simulink model "sampleModel1734_sub"  (R2023a)
settings: Solver=VariableStepAuto  StartTime=0.0  StopTime=10.0  RelTol=1e-3
libraries: hdlsllib x3
settings Model: Creator=user1  LastModifiedBy=user1
settings OptimizationCC: BlockReduction=off  ConditionallyExecuteInputs=off

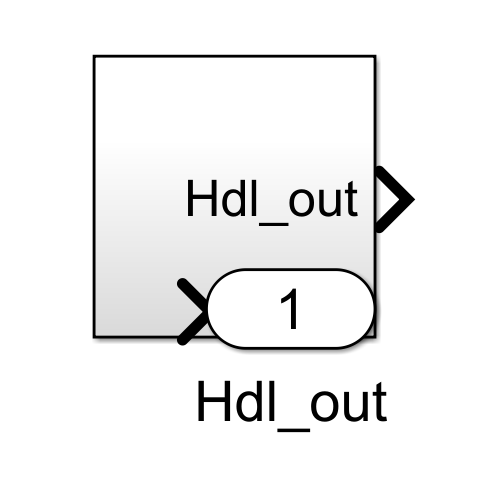
[thumbnail: Simulink's stored preview of the top-level diagram]
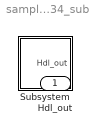
== system sampleModel1734_sub ==
  Subsystem : Subsystem
  Hdl_out : Outport  OutDataTypeStr=uint8

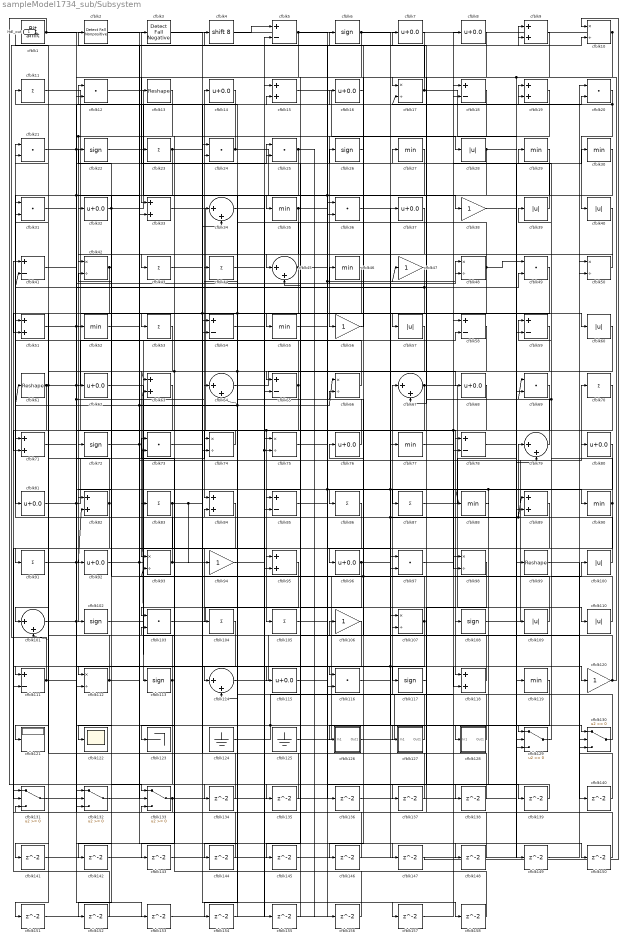
== system sampleModel1734_sub/Subsystem ==
  cfblk1 : hdlsllib/Logic and Bit Operations/Bit Shift  mode=Shift Left Logical  N=0
  cfblk{10,17,42,48,50,66,74..75,93,98,107,112} (12 alike) : Product  Inputs=*/  OutDataTypeStr=uint8  RndMeth=Zero  SaturateOnIntegerOverflow=on
  cfblk{28,39..40,57,60,100,109..110} (8 alike) : Abs  OutDataTypeStr=uint8  SaturateOnIntegerOverflow=off
  cfblk{34,45,64,67,79,101,114} (7 alike) : Sum  Inputs=|++  OutDataTypeStr=uint8
  cfblk{6,22,26,72,102,108,113,117} (8 alike) : Signum
  cfblk{12,20..21,24..25,31,36,49,69,73,97,103,116} (13 alike) : DotProduct  OutDataTypeStr=uint8
  cfblk{11,23,43..44,53,70,83,86..87,91,104..105} (12 alike) : Sum  Inputs=+  OutDataTypeStr=uint8
  cfblk{38,47,56,94,106,120} (6 alike) : Gain  OutDataTypeStr=uint8
  cfblk{5,18,41,54,58..59,65,78,85,111} (10 alike) : Sum  Inputs=+-  OutDataTypeStr=uint8
  cfblk{7..8,14,16,32,37,62,68,76,80..81,92,96,115} (14 alike) : Bias  Bias=0.0  SaturateOnIntegerOverflow=off
  cfblk{9,15,19,33,51,63,71,82,84,89,95,118} (12 alike) : Sum  OutDataTypeStr=uint8
  cfblk{27,29..30,35,46,52,55,77,88,90,119} (11 alike) : MinMax  OutDataTypeStr=uint8
  cfblk121 : Display
  cfblk122 : Scope
  cfblk123 : Terminator
  cfblk124 : Ground
  cfblk125 : Ground
  cfblk126 : Subsystem
      settings: LibrarySourceBlock=|
      | hdlsllib/Ports &
      | Subsystems/Subsystem
  cfblk127 : Subsystem
      settings: LibrarySourceBlock=|
      | hdlsllib/Ports &
      | Subsystems/Subsystem
  cfblk128 : Subsystem
      settings: LibrarySourceBlock=|
      | hdlsllib/Ports &
      | Subsystems/Subsystem
  cfblk{129..133} (5 alike) : Switch  OutDataTypeStr=uint8  SaturateOnIntegerOverflow=off  InputSameDT=off
  cfblk13 : Reshape
  cfblk{134..158} (25 alike) : Delay  SampleTime=1
  cfblk2 : hdlsllib/Logic and Bit Operations/Detect Fall Nonpositive  vinit=0  OutDataTypeStr=uint8
  cfblk3 : hdlsllib/Logic and Bit Operations/Detect Fall Negative  vinit=0  OutDataTypeStr=uint8
  cfblk4 : ArithShift  BitShiftNumber=8
  cfblk61 : Reshape
  cfblk99 : Reshape
  Hdl_out : Outport  OutDataTypeStr=uint8
  wires:
  cfblk100/1 -> cfblk42/2, cfblk79/1
  cfblk69/1 -> cfblk85/2, cfblk105/1
  cfblk89/1 -> cfblk91/1
  cfblk12/1 -> cfblk38/1
  cfblk63/1 -> cfblk102/1
  cfblk59/1 -> cfblk154/1, cfblk113/1
  cfblk13/1 -> cfblk72/1
  cfblk66/1 -> cfblk14/1
  cfblk108/1 -> cfblk70/1
  cfblk120/1 -> cfblk25/2, cfblk17/1
  cfblk15/1 -> cfblk28/1
  cfblk11/1 -> cfblk55/1
  cfblk67/1 -> cfblk122/1, cfblk110/1
  cfblk32/1 -> cfblk52/1, cfblk16/1
  cfblk96/1 -> cfblk135/1, cfblk130/3
  cfblk111/1 -> cfblk15/2, cfblk4/1
  cfblk130/1 -> cfblk67/1
  cfblk21/1 -> cfblk115/1, cfblk118/1
  cfblk46/1 -> cfblk53/1
  cfblk38/1 -> cfblk99/1
  cfblk64/1 -> cfblk68/1
  cfblk14/1 -> cfblk132/3, cfblk32/1
  cfblk110/1 -> cfblk39/1, cfblk69/1
  cfblk9/1 -> cfblk129/3, cfblk86/1
  cfblk65/1 -> cfblk31/2, cfblk84/1
  cfblk1/1 -> cfblk133/1, cfblk33/2, cfblk130/1
  cfblk26/1 -> cfblk96/1
  cfblk33/1 -> cfblk78/1
  cfblk62/1 -> cfblk117/1
  cfblk109/1 -> cfblk22/1
  cfblk81/1 -> cfblk83/1, cfblk34/1
  cfblk116/1 -> cfblk48/2, cfblk89/1
  cfblk50/1 -> cfblk45/1
  cfblk22/1 -> cfblk24/2
  cfblk93/1 -> cfblk157/1, cfblk21/1
  cfblk103/1 -> cfblk108/1
  cfblk18/1 -> cfblk56/1
  cfblk76/1 -> cfblk44/1
  cfblk71/1 -> cfblk64/1
  cfblk54/1 -> cfblk120/1, cfblk75/2
  cfblk23/1 -> cfblk158/1, cfblk81/1
  cfblk19/1 -> cfblk103/1
  cfblk17/1 -> cfblk109/1, cfblk2/1
  cfblk51/1 -> cfblk78/2, cfblk74/1
  cfblk37/1 -> cfblk42/1
  cfblk56/1 -> cfblk6/1
  cfblk92/1 -> cfblk19/2, cfblk34/2
  cfblk27/1 -> cfblk35/1
  cfblk53/1 -> cfblk82/1
  cfblk86/1 -> cfblk104/1
  cfblk20/1 -> cfblk17/2, cfblk40/1
  cfblk117/1 -> cfblk7/1
  cfblk125/1 -> cfblk8/1
  cfblk79/1 -> cfblk26/1
  cfblk101/1 -> cfblk148/1, cfblk46/1
  cfblk41/1 -> cfblk25/1
  cfblk90/1 -> cfblk92/1, cfblk27/1
  cfblk39/1 -> cfblk3/1
  cfblk57/1 -> cfblk93/1
  cfblk102/1 -> cfblk106/1
  cfblk126/1(Out1) -> cfblk98/1
  cfblk4/1 -> cfblk5/1
  cfblk2/1 -> cfblk95/1
  cfblk87/1 -> cfblk30/1
  cfblk82/1 -> cfblk21/2, cfblk121/1
  cfblk61/1 -> cfblk71/2, cfblk101/2, cfblk147/1, cfblk37/1
  cfblk42/1 -> cfblk62/1, cfblk111/1
  cfblk95/1 -> cfblk123/1
  cfblk36/1 -> cfblk107/1
  cfblk10/1 -> Hdl_out/1, cfblk65/1
  cfblk45/1 -> cfblk13/1, cfblk51/2, cfblk19/1
  cfblk128/1(Out1) -> cfblk61/1, cfblk64/2
  cfblk97/1 -> cfblk10/2
  cfblk16/1 -> cfblk116/1
  cfblk132/1 -> cfblk80/1
  cfblk127/1(Out1) -> cfblk11/1
  cfblk52/1 -> cfblk90/1
  cfblk94/1 -> cfblk48/1
  cfblk72/1 -> cfblk150/1, cfblk66/1, cfblk9/1
  cfblk114/1 -> cfblk50/2
  cfblk80/1 -> cfblk128/1(In1), cfblk116/2
  cfblk113/1 -> cfblk152/1, cfblk31/1
  cfblk28/1 -> cfblk142/1, cfblk119/1
  cfblk119/1 -> cfblk126/1(In1)
  cfblk91/1 -> cfblk82/2, cfblk49/2, cfblk63/2
  cfblk35/1 -> cfblk129/1, cfblk43/1
  cfblk70/1 -> cfblk132/2, cfblk98/2
  cfblk129/1 -> cfblk59/1
  cfblk133/1 -> cfblk131/3, cfblk18/1
  cfblk124/1 -> cfblk129/2, cfblk58/1
  cfblk49/1 -> cfblk144/1, cfblk143/1, cfblk63/1
  cfblk29/1 -> cfblk67/2
  cfblk77/1 -> cfblk29/1
  cfblk105/1 -> cfblk9/2, cfblk47/1
  cfblk118/1 -> cfblk76/1
  cfblk73/1 -> cfblk20/2
  cfblk3/1 -> cfblk87/1
  cfblk30/1 -> cfblk95/2
  cfblk106/1 -> cfblk111/2
  cfblk131/1 -> cfblk73/1
  cfblk5/1 -> cfblk12/2, cfblk139/1, cfblk88/1
  cfblk48/1 -> cfblk145/1, cfblk49/1, cfblk12/1
  cfblk44/1 -> cfblk5/2
  cfblk47/1 -> cfblk41/2, cfblk85/1
  cfblk7/1 -> cfblk33/1
  cfblk8/1 -> cfblk57/1
  cfblk83/1 -> cfblk112/2, cfblk94/1, cfblk74/2
  cfblk24/1 -> cfblk23/1, cfblk77/1, cfblk36/2
  cfblk75/1 -> cfblk97/2
  cfblk6/1 -> cfblk54/2, cfblk89/2, cfblk118/2, cfblk130/2
  cfblk25/1 -> cfblk156/1, cfblk114/1
  cfblk74/1 -> cfblk71/1
  cfblk55/1 -> cfblk60/1
  cfblk107/1 -> cfblk112/1, cfblk93/2, cfblk66/2
  cfblk112/1 -> cfblk51/1, cfblk100/1
  cfblk60/1 -> cfblk101/1
  cfblk84/1 -> cfblk131/2
  cfblk43/1 -> cfblk59/2, cfblk127/1(In1)
  cfblk115/1 -> cfblk58/2
  cfblk40/1 -> cfblk134/1
  cfblk134/1 -> cfblk1/1
  cfblk135/1 -> cfblk24/1
  cfblk85/1 -> cfblk136/1
  cfblk136/1 -> cfblk69/2
  cfblk98/1 -> cfblk137/1
  cfblk137/1 -> cfblk84/2
  cfblk88/1 -> cfblk138/1
  cfblk138/1 -> cfblk54/1
  cfblk139/1 -> cfblk133/2
  cfblk99/1 -> cfblk140/1
  cfblk140/1 -> cfblk20/1
  cfblk58/1 -> cfblk141/1
  cfblk141/1 -> cfblk97/1
  cfblk142/1 -> cfblk15/1
  cfblk143/1 -> cfblk65/2
  cfblk144/1 -> cfblk103/2
  cfblk145/1 -> cfblk79/2
  cfblk68/1 -> cfblk146/1
  cfblk146/1 -> cfblk132/1
  cfblk147/1 -> cfblk10/1
  cfblk148/1 -> cfblk107/2
  cfblk78/1 -> cfblk149/1
  cfblk149/1 -> cfblk50/1
  cfblk150/1 -> cfblk41/1
  cfblk104/1 -> cfblk151/1
  cfblk151/1 -> cfblk75/1
  cfblk152/1 -> cfblk131/1
  cfblk31/1 -> cfblk153/1
  cfblk153/1 -> cfblk36/1
  cfblk154/1 -> cfblk114/2
  cfblk34/1 -> cfblk155/1
  cfblk155/1 -> cfblk45/2
  cfblk156/1 -> cfblk133/3
  cfblk157/1 -> cfblk18/2
  cfblk158/1 -> cfblk73/2

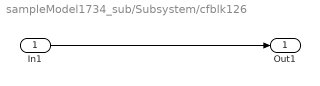
== system sampleModel1734_sub/Subsystem/cfblk126 ==
  In1 : Inport
  Out1 : Outport
  wires:
  In1/1 -> Out1/1

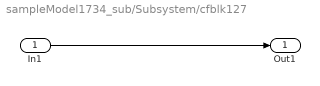
== system sampleModel1734_sub/Subsystem/cfblk127 ==
  In1 : Inport
  Out1 : Outport
  wires:
  In1/1 -> Out1/1

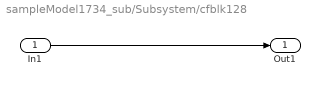
== system sampleModel1734_sub/Subsystem/cfblk128 ==
  In1 : Inport
  Out1 : Outport
  wires:
  In1/1 -> Out1/1
